simulink model "OilP_DD"  (R2016b)
settings: configuration reference "CodeGenConfigSet" (kept outside this file)
values from neighbouring files (symbols this model uses):
  Oil_pAnaHi_C = Calibration.Parameter    [init_OilP_DD.m]    (also in init_OilP_DD_SIL.m = Simulink.Parameter)
  Oil_pMaxP_CUR = Calibration.Parameter    [init_OilP_DD.m]    (also in init_OilP_DD_SIL.m = Simulink.Parameter)
  Oil_pMaxP_CURX = Calibration.Parameter    [init_OilP_DD.m]    (also in init_OilP_DD_SIL.m = Simulink.Parameter)
  Oil_pMinP_CUR = Calibration.Parameter    [init_OilP_DD.m]    (also in init_OilP_DD_SIL.m = Simulink.Parameter)
  Oil_pMinP_CURX = Calibration.Parameter    [init_OilP_DD.m]    (also in init_OilP_DD_SIL.m = Simulink.Parameter)
  Oil_pTransfPSwmp_CUR = Calibration.Parameter    [init_OilP_DD.m]    (also in init_OilP_DD_SIL.m = Simulink.Parameter)
  Oil_pTransfPSwmp_CURX = Calibration.Parameter    [init_OilP_DD.m]    (also in init_OilP_DD_SIL.m = Simulink.Parameter)
  Oil_tiPhysRngHiPSwmpDefDeb_C = Calibration.Parameter    [init_OilP_DD.m]    (also in init_OilP_DD_SIL.m = Simulink.Parameter)
  Oil_tiPhysRngHiPSwmpOKDeb_C = Calibration.Parameter    [init_OilP_DD.m]    (also in init_OilP_DD_SIL.m = Simulink.Parameter)
  Oil_tiPhysRngLoPSwmpDefDeb_C = Calibration.Parameter    [init_OilP_DD.m]    (also in init_OilP_DD_SIL.m = Simulink.Parameter)
  Oil_tiPhysRngLoPSwmpOKDeb_C = Calibration.Parameter    [init_OilP_DD.m]    (also in init_OilP_DD_SIL.m = Simulink.Parameter)
  Oil_tiSRCMaxPSwmpDefDeb_C = Calibration.Parameter    [init_OilP_DD.m]    (also in init_OilP_DD_SIL.m = Simulink.Parameter)
  Oil_tiSRCMaxPSwmpOKDeb_C = Calibration.Parameter    [init_OilP_DD.m]    (also in init_OilP_DD_SIL.m = Simulink.Parameter)
  Oil_tiSRCMinPSwmpDefDeb_C = Calibration.Parameter    [init_OilP_DD.m]    (also in init_OilP_DD_SIL.m = Simulink.Parameter)
  Oil_tiSRCMinPSwmpOKDeb_C = Calibration.Parameter    [init_OilP_DD.m]    (also in init_OilP_DD_SIL.m = Simulink.Parameter)
  Oil_tLimP_C = Calibration.Parameter    [init_OilP_DD.m]    (also in init_OilP_DD_SIL.m = Simulink.Parameter)
  Oil_uSRCPSwmpMax_C = Calibration.Parameter    [init_OilP_DD.m]    (also in init_OilP_DD_SIL.m = Simulink.Parameter)
  Oil_uSRCPSwmpMin_C = Calibration.Parameter    [init_OilP_DD.m]    (also in init_OilP_DD_SIL.m = Simulink.Parameter)
  OilP_tiPlusDebHiLo_C = Calibration.Parameter    [init_OilP_DD.m]    (also in init_OilP_DD_SIL.m = Simulink.Parameter)
  OilP_tiPlusDebLoHi_C = Calibration.Parameter    [init_OilP_DD.m]    (also in init_OilP_DD_SIL.m = Simulink.Parameter)
undefined symbols (not defined in the file or in its folder): CEngDsT_tTransf_CURX, OilP_DD_DT
libraries: CXLib x13
settings Model: Creator=Wollf  LastModifiedBy=xinchangran
settings ConfigSetRef: SourceLocation=Base Workspace

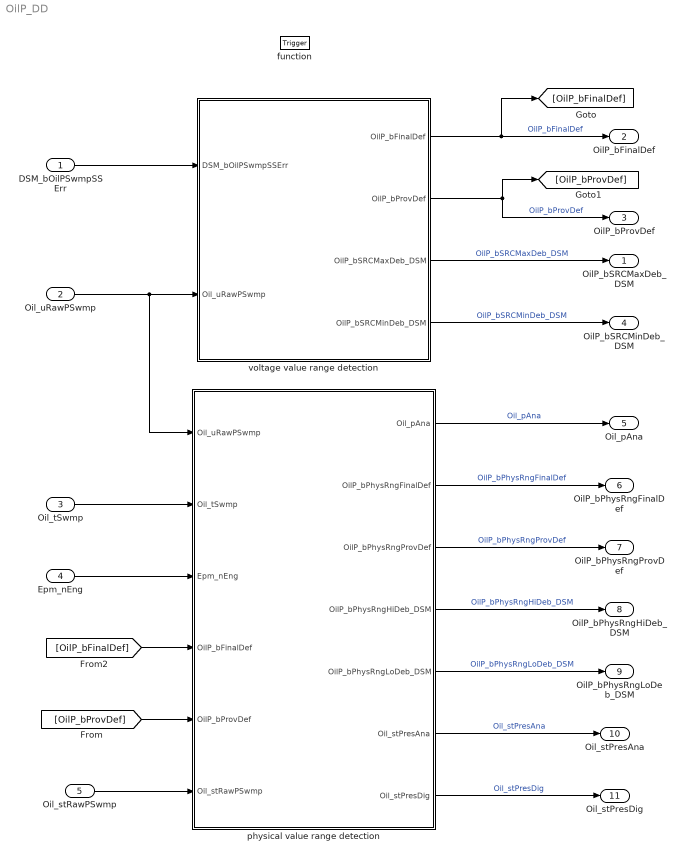
== system OilP_DD ==
  DSM_bOilPSwmpSSErr : Inport  Description=state of FId_OilPSwmpSSErr  OutMin=0  OutMax=1  OutDataTypeStr=boolean
  Oil_uRawPSwmp : Inport  Tag=mv  Description=Raw value of voltage from the ADC  Port=2  OutMin=0  OutMax=5000  OutDataTypeStr=Ad_mv
  Oil_tSwmp : Inport  Tag=deg  Description=Oil temperature in oil sump  Port=3  OutMin=-50  OutMax=200  OutDataTypeStr=Temp_deg
  Epm_nEng : Inport  Tag=rpm  Description=Engine speed  Port=4  OutMin=0  OutMax=6000  OutDataTypeStr=EngSpeed_rpm
  Oil_stRawPSwmp : Inport  Description=the digital sensor raw voltage value  Port=5  OutMin=0  OutMax=1  OutDataTypeStr=boolean
  function : TriggerPort  TriggerType=function-call  VariantControl=Variant
  " voltage value range detection" : Subsystem
  physical value range detection : Subsystem
  OilP_bSRCMaxDeb_DSM : Outport  Description=status of OilP_bSRCMaxDeb  OutMin=0  OutMax=1  OutDataTypeStr=boolean
  OilP_bFinalDef : Outport  Description=Status sensor of the oil pressure finally defect  Port=2  OutMin=0  OutMax=1  OutDataTypeStr=boolean
  OilP_bProvDef : Outport  Description=Status sensor of the oil pressure temporary defect  Port=3  OutMin=0  OutMax=1  OutDataTypeStr=boolean
  OilP_bSRCMinDeb_DSM : Outport  Description=status of OilP_bSRCMinDeb  Port=4  OutMin=0  OutMax=1  OutDataTypeStr=boolean
  Oil_pAna : Outport  Tag=kPa  Description=Oil pressure for analog input  Port=5  OutMin=0  OutMax=1200  OutDataTypeStr=AirPressure_kPa
  OilP_bPhysRngFinalDef : Outport  Description=Status sensor of the oil pressure physical signal range check finally defect  Port=6  OutMin=0  OutMax=1  OutDataTypeStr=boolean
  OilP_bPhysRngProvDef : Outport  Description=Status sensor of the oil pressure physical signal range check temporary defect  Port=7  OutMin=0  OutMax=1  OutDataTypeStr=boolean
  OilP_bPhysRngHiDeb_DSM : Outport  Description=status of OilP_bPhysRngHiDeb  Port=8  OutMin=0  OutMax=1  OutDataTypeStr=boolean
  OilP_bPhysRngLoDeb_DSM : Outport  Description=status of OilP_bPhysRngHiDeb  Port=9  OutMin=0  OutMax=1  OutDataTypeStr=boolean
  Oil_stPresAna : Outport  Description=Oil pressure status for analog input  Port=10  OutMin=0  OutMax=1  OutDataTypeStr=boolean
  Oil_stPresDig : Outport  Description=Oil pressure status for digital input  Port=11  OutMin=0  OutMax=1  OutDataTypeStr=boolean
  wires:
  Oil_uRawPSwmp/1 -> physical value range detection/1(Oil_uRawPSwmp), " voltage value range detection"/2(Oil_uRawPSwmp)
  DSM_bOilPSwmpSSErr/1 -> " voltage value range detection"/1(DSM_bOilPSwmpSSErr)
  " voltage value range detection"/1(OilP_bFinalDef) -> OilP_bFinalDef/1, [OilP_bFinalDef]  "OilP_bFinalDef"
  " voltage value range detection"/2(OilP_bProvDef) -> OilP_bProvDef/1, [OilP_bProvDef]  "OilP_bProvDef"
  " voltage value range detection"/3(OilP_bSRCMaxDeb_DSM) -> OilP_bSRCMaxDeb_DSM/1  "OilP_bSRCMaxDeb_DSM"
  " voltage value range detection"/4(OilP_bSRCMinDeb_DSM) -> OilP_bSRCMinDeb_DSM/1  "OilP_bSRCMinDeb_DSM"
  Oil_tSwmp/1 -> physical value range detection/2(Oil_tSwmp)
  Epm_nEng/1 -> physical value range detection/3(Epm_nEng)
  physical value range detection/1(Oil_pAna) -> Oil_pAna/1  "Oil_pAna"
  physical value range detection/2(OilP_bPhysRngFinalDef) -> OilP_bPhysRngFinalDef/1  "OilP_bPhysRngFinalDef"
  physical value range detection/3(OilP_bPhysRngProvDef) -> OilP_bPhysRngProvDef/1  "OilP_bPhysRngProvDef"
  physical value range detection/4(OilP_bPhysRngHiDeb_DSM) -> OilP_bPhysRngHiDeb_DSM/1  "OilP_bPhysRngHiDeb_DSM"
  physical value range detection/5(OilP_bPhysRngLoDeb_DSM) -> OilP_bPhysRngLoDeb_DSM/1  "OilP_bPhysRngLoDeb_DSM"
  [OilP_bFinalDef] -> physical value range detection/4(OilP_bFinalDef)
  [OilP_bProvDef] -> physical value range detection/5(OilP_bProvDef)
  physical value range detection/6(Oil_stPresAna) -> Oil_stPresAna/1  "Oil_stPresAna"
  physical value range detection/7(Oil_stPresDig) -> Oil_stPresDig/1  "Oil_stPresDig"
  Oil_stRawPSwmp/1 -> physical value range detection/6(Oil_stRawPSwmp)

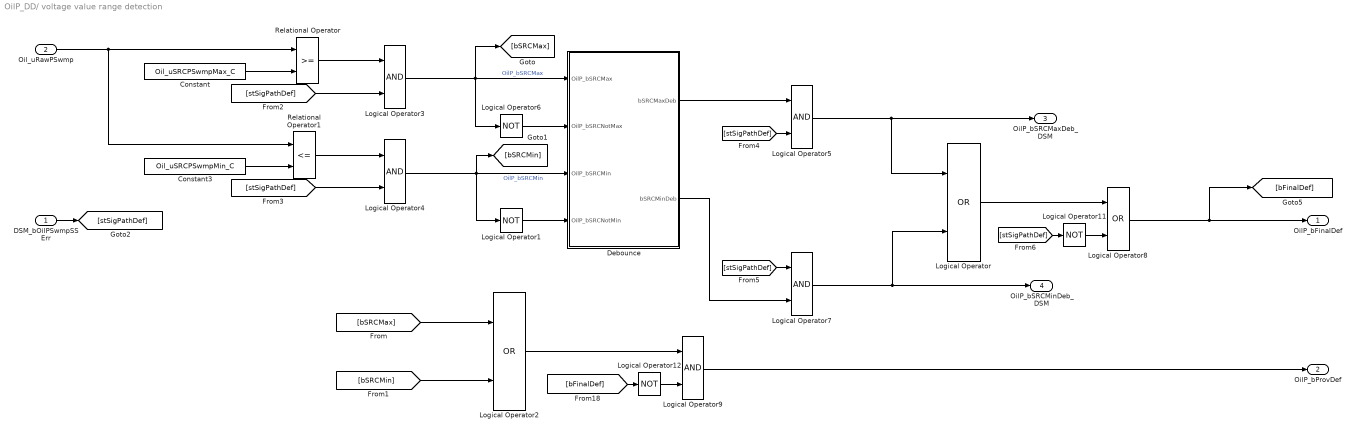
== system OilP_DD/ voltage value range detection ==
  DSM_bOilPSwmpSSErr : Inport
  Oil_uRawPSwmp : Inport  Port=2
  Constant : Constant  Value=Oil_uSRCPSwmpMax_C
  Constant3 : Constant  Value=Oil_uSRCPSwmpMin_C
  Debounce : Subsystem
  Logical Operator : Logic  Operator=OR  AllPortsSameDT=off  OutDataTypeStr=boolean
  Logical Operator{1,6,11..12} (4 alike) : Logic  Operator=NOT  AllPortsSameDT=off  OutDataTypeStr=boolean
  Logical Operator2 : Logic  Operator=OR  AllPortsSameDT=off  OutDataTypeStr=boolean
  Logical Operator{3..5,7,9} (5 alike) : Logic  AllPortsSameDT=off  OutDataTypeStr=boolean
  Logical Operator8 : Logic  Operator=OR  AllPortsSameDT=off  OutDataTypeStr=boolean
  Relational Operator : RelationalOperator  OutDataTypeStr=boolean  RndMeth=Nearest  InputSameDT=on
  Relational Operator1 : RelationalOperator  Operator=<=  OutDataTypeStr=boolean  RndMeth=Nearest  InputSameDT=on
  OilP_bFinalDef : Outport
  OilP_bProvDef : Outport  Port=2
  OilP_bSRCMaxDeb_DSM : Outport  Port=3
  OilP_bSRCMinDeb_DSM : Outport  Port=4
  wires:
  Oil_uRawPSwmp/1 -> Relational Operator1/1, Relational Operator/1
  Relational Operator1/1 -> Logical Operator4/1
  [stSigPathDef] -> Logical Operator3/2
  Logical Operator1/1 -> Debounce/4(OilP_bSRCNotMin)
  Logical Operator12/1 -> Logical Operator9/2
  Debounce/1(bSRCMaxDeb) -> Logical Operator5/1
  Constant/1 -> Relational Operator/2
  [bSRCMin] -> Logical Operator2/2
  Logical Operator4/1 -> [bSRCMin], Debounce/3(OilP_bSRCMin), Logical Operator1/1  "OilP_bSRCMin"
  Logical Operator5/1 -> OilP_bSRCMaxDeb_DSM/1, Logical Operator/1
  [stSigPathDef] -> Logical Operator4/2
  Logical Operator8/1 -> OilP_bFinalDef/1, [bFinalDef]
  Logical Operator7/1 -> OilP_bSRCMinDeb_DSM/1, Logical Operator/2
  Logical Operator9/1 -> OilP_bProvDef/1
  Relational Operator/1 -> Logical Operator3/1
  Logical Operator11/1 -> Logical Operator8/2
  [stSigPathDef] -> Logical Operator5/2
  Logical Operator2/1 -> Logical Operator9/1
  [bSRCMax] -> Logical Operator2/1
  Logical Operator3/1 -> [bSRCMax], Logical Operator6/1, Debounce/1(OilP_bSRCMax)  "OilP_bSRCMax"
  [bFinalDef] -> Logical Operator12/1
  Logical Operator6/1 -> Debounce/2(OilP_bSRCNotMax)
  Debounce/2(bSRCMinDeb) -> Logical Operator7/2
  [stSigPathDef] -> Logical Operator11/1
  Logical Operator/1 -> Logical Operator8/1
  [stSigPathDef] -> Logical Operator7/1
  Constant3/1 -> Relational Operator1/2
  DSM_bOilPSwmpSSErr/1 -> [stSigPathDef]

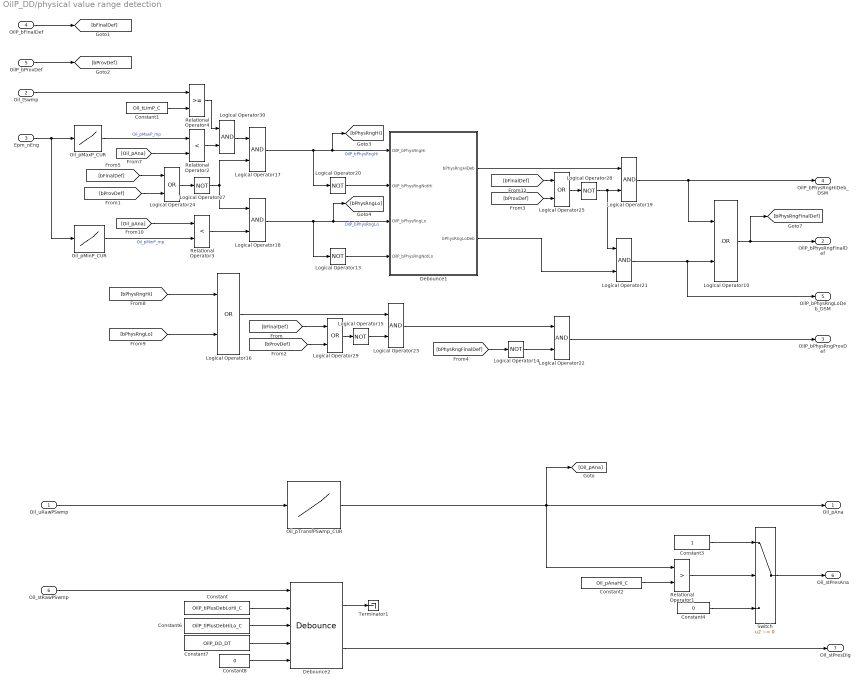
== system OilP_DD/physical value range detection ==
  Oil_uRawPSwmp : Inport
  Oil_tSwmp : Inport  Port=2
  Epm_nEng : Inport  Port=3
  OilP_bFinalDef : Inport  Port=4
  OilP_bProvDef : Inport  Port=5
  Oil_stRawPSwmp : Inport  Port=6
  Constant : Constant  Value=OilP_tiPlusDebLoHi_C
  Constant1 : Constant  Value=Oil_tLimP_C  SampleTime=-1
  Constant2 : Constant  Value=Oil_pAnaHi_C
  Constant3 : Constant  OutDataTypeStr=Inherit: Inherit via back propagation
  Constant4 : Constant  Value=0  OutDataTypeStr=Inherit: Inherit via back propagation
  Constant6 : Constant  Value=OilP_tiPlusDebHiLo_C
  Constant7 : Constant  Value=OilP_DD_DT
  Constant8 : Constant  Value=0  OutDataTypeStr=Inherit: Inherit via back propagation
  Debounce1 : Subsystem
  Debounce2 : CXLib/Debounce
  Logical Operator10 : Logic  Operator=OR  AllPortsSameDT=off  OutDataTypeStr=boolean
  Logical Operator{13..15,20,27..28} (6 alike) : Logic  Operator=NOT  AllPortsSameDT=off  OutDataTypeStr=boolean
  Logical Operator16 : Logic  Operator=OR  AllPortsSameDT=off  OutDataTypeStr=boolean
  Logical Operator{17..19,21..23} (6 alike) : Logic  AllPortsSameDT=off  OutDataTypeStr=boolean
  Logical Operator24 : Logic  Operator=OR  OutDataTypeStr=boolean
  Logical Operator25 : Logic  Operator=OR  OutDataTypeStr=boolean
  Logical Operator29 : Logic  Operator=OR  OutDataTypeStr=boolean
  Logical Operator30 : Logic  OutDataTypeStr=boolean
  Oil_pMaxP_CUR : Lookup_n-D  DialogController=Simulink.DDGSource  NumberOfTableDimensions=1  BreakpointsForDimension1=Oil_pMaxP_CURX  BreakpointsForDimension2=CEngDsT_tTransf_CURX  IndexSearchMethod=Linear search  BeginIndexSearchUsingPreviousIndexResult=on  Table=Oil_pMaxP_CUR  ExtrapMethod=Clip  UseLastTableValue=on  InternalRulePriority=Speed  OutDataTypeStr=Inherit: Inherit via back propagation  SaturateOnIntegerOverflow=on
  Oil_pMinP_CUR : Lookup_n-D  DialogController=Simulink.DDGSource  NumberOfTableDimensions=1  BreakpointsForDimension1=Oil_pMinP_CURX  BreakpointsForDimension2=CEngDsT_tTransf_CURX  IndexSearchMethod=Linear search  BeginIndexSearchUsingPreviousIndexResult=on  Table=Oil_pMinP_CUR  ExtrapMethod=Clip  UseLastTableValue=on  InternalRulePriority=Speed  OutDataTypeStr=Inherit: Inherit via back propagation  SaturateOnIntegerOverflow=on
  Oil_pTransfPSwmp_CUR : Lookup_n-D  DialogController=Simulink.DDGSource  NumberOfTableDimensions=1  BreakpointsForDimension1=Oil_pTransfPSwmp_CURX  BreakpointsForDimension2=CEngDsT_tTransf_CURX  IndexSearchMethod=Linear search  BeginIndexSearchUsingPreviousIndexResult=on  Table=Oil_pTransfPSwmp_CUR  ExtrapMethod=Clip  UseLastTableValue=on  InternalRulePriority=Speed  OutDataTypeStr=Inherit: Inherit via back propagation  SaturateOnIntegerOverflow=on
  Relational Operator1 : RelationalOperator  Operator=>  OutDataTypeStr=boolean  RndMeth=Nearest  InputSameDT=on
  Relational Operator2 : RelationalOperator  Operator=<  OutDataTypeStr=boolean  RndMeth=Nearest  InputSameDT=on
  Relational Operator3 : RelationalOperator  Operator=<  OutDataTypeStr=boolean  RndMeth=Nearest  InputSameDT=on
  Relational Operator4 : RelationalOperator  OutDataTypeStr=boolean  RndMeth=Nearest  InputSameDT=on
  Switch : Switch  Criteria=u2 ~= 0  InputSameDT=on
  Terminator1 : Terminator
  Oil_pAna : Outport
  OilP_bPhysRngFinalDef : Outport  Port=2
  OilP_bPhysRngProvDef : Outport  Port=3
  OilP_bPhysRngHiDeb_DSM : Outport  Port=4
  OilP_bPhysRngLoDeb_DSM : Outport  Port=5
  Oil_stPresAna : Outport  Port=6
  Oil_stPresDig : Outport  Port=7
  wires:
  Logical Operator17/1 -> Logical Operator20/1, Debounce1/1(OilP_bPhysRngHi), [bPhysRngHi]  "OilP_bPhysRngHi"
  Logical Operator18/1 -> Logical Operator13/1, [bPhysRngLo], Debounce1/3(OilP_bPhysRngLo)  "OilP_bPhysRngLo"
  Oil_pMinP_CUR/1 -> Relational Operator3/2  "Oil_pMinP_mp"
  [bPhysRngHi] -> Logical Operator16/1
  [bPhysRngLo] -> Logical Operator16/2
  Logical Operator24/1 -> Logical Operator27/1
  Logical Operator21/1 -> OilP_bPhysRngLoDeb_DSM/1, Logical Operator10/2
  Logical Operator22/1 -> OilP_bPhysRngProvDef/1
  Relational Operator4/1 -> Logical Operator30/1
  Logical Operator28/1 -> Logical Operator21/1, Logical Operator19/2
  Logical Operator20/1 -> Debounce1/2(OilP_bPhysRngNotHi)
  [bProvDef] -> Logical Operator24/2
  Logical Operator29/1 -> Logical Operator15/1
  [bFinalDef] -> Logical Operator24/1
  Epm_nEng/1 -> Oil_pMinP_CUR/1, Oil_pMaxP_CUR/1
  Relational Operator2/1 -> Logical Operator30/2
  Logical Operator10/1 -> OilP_bPhysRngFinalDef/1, [bPhysRngFinalDef]
  Logical Operator30/1 -> Logical Operator17/1
  Debounce1/2(bPhysRngLoDeb) -> Logical Operator21/2
  Constant1/1 -> Relational Operator4/2
  [bPhysRngFinalDef] -> Logical Operator14/1
  [bProvDef] -> Logical Operator25/2
  Logical Operator14/1 -> Logical Operator22/2
  [bFinalDef] -> Logical Operator29/1
  Oil_tSwmp/1 -> Relational Operator4/1
  [bFinalDef] -> Logical Operator25/1
  Logical Operator25/1 -> Logical Operator28/1
  Oil_pMaxP_CUR/1 -> Relational Operator2/1  "Oil_pMaxP_mp"
  [bProvDef] -> Logical Operator29/2
  Logical Operator27/1 -> Logical Operator18/1, Logical Operator17/2
  Logical Operator23/1 -> Logical Operator22/1
  Logical Operator16/1 -> Logical Operator23/1
  Logical Operator15/1 -> Logical Operator23/2
  Debounce1/1(bPhysRngHiDeb) -> Logical Operator19/1
  Relational Operator3/1 -> Logical Operator18/2
  Logical Operator13/1 -> Debounce1/4(OilP_bPhysRngNotLo)
  Oil_uRawPSwmp/1 -> Oil_pTransfPSwmp_CUR/1
  OilP_bProvDef/1 -> [bProvDef]
  OilP_bFinalDef/1 -> [bFinalDef]
  [Oil_pAna] -> Relational Operator2/2
  [Oil_pAna] -> Relational Operator3/1
  Constant2/1 -> Relational Operator1/2
  Relational Operator1/1 -> Switch/2
  Constant3/1 -> Switch/1
  Constant4/1 -> Switch/3
  Switch/1 -> Oil_stPresAna/1
  Constant6/1 -> Debounce2/3
  Debounce2/1 -> Terminator1/1
  Constant/1 -> Debounce2/2
  Constant7/1 -> Debounce2/4
  Constant8/1 -> Debounce2/5
  Oil_stRawPSwmp/1 -> Debounce2/1
  Debounce2/2 -> Oil_stPresDig/1
  Oil_pTransfPSwmp_CUR/1 -> [Oil_pAna], Oil_pAna/1, Relational Operator1/1
  Logical Operator19/1 -> OilP_bPhysRngHiDeb_DSM/1, Logical Operator10/1

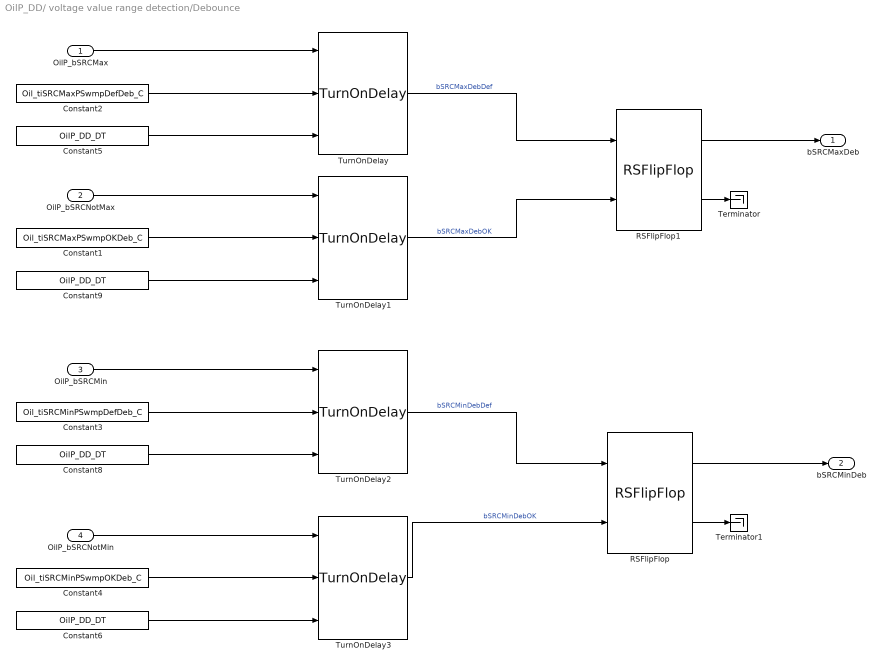
== system OilP_DD/ voltage value range detection/Debounce ==
  OilP_bSRCMax : Inport
  OilP_bSRCNotMax : Inport  Port=2
  OilP_bSRCMin : Inport  Port=3
  OilP_bSRCNotMin : Inport  Port=4
  Constant1 : Constant  Value=Oil_tiSRCMaxPSwmpOKDeb_C
  Constant2 : Constant  Value=Oil_tiSRCMaxPSwmpDefDeb_C
  Constant3 : Constant  Value=Oil_tiSRCMinPSwmpDefDeb_C
  Constant4 : Constant  Value=Oil_tiSRCMinPSwmpOKDeb_C
  Constant{5..6,8..9} (4 alike) : Constant  Value=OilP_DD_DT  OutDataTypeStr=Inherit: Inherit via back propagation
  RSFlipFlop : CXLib/RSFlipFlop
  RSFlipFlop1 : CXLib/RSFlipFlop
  Terminator : Terminator
  Terminator1 : Terminator
  TurnOnDelay{,1..3} (4 alike) : CXLib/TurnOnDelay
  bSRCMaxDeb : Outport
  bSRCMinDeb : Outport  Port=2
  wires:
  RSFlipFlop/1 -> bSRCMinDeb/1
  RSFlipFlop1/1 -> bSRCMaxDeb/1
  TurnOnDelay1/1 -> RSFlipFlop1/2  "bSRCMaxDebOK"
  Constant3/1 -> TurnOnDelay2/2
  Constant1/1 -> TurnOnDelay1/2
  Constant2/1 -> TurnOnDelay/2
  TurnOnDelay/1 -> RSFlipFlop1/1  "bSRCMaxDebDef"
  OilP_bSRCNotMax/1 -> TurnOnDelay1/1
  OilP_bSRCMin/1 -> TurnOnDelay2/1
  TurnOnDelay2/1 -> RSFlipFlop/1  "bSRCMinDebDef"
  OilP_bSRCNotMin/1 -> TurnOnDelay3/1
  TurnOnDelay3/1 -> RSFlipFlop/2  "bSRCMinDebOK"
  Constant4/1 -> TurnOnDelay3/2
  RSFlipFlop1/2 -> Terminator/1
  RSFlipFlop/2 -> Terminator1/1
  OilP_bSRCMax/1 -> TurnOnDelay/1
  Constant5/1 -> TurnOnDelay/3
  Constant8/1 -> TurnOnDelay2/3
  Constant6/1 -> TurnOnDelay3/3
  Constant9/1 -> TurnOnDelay1/3

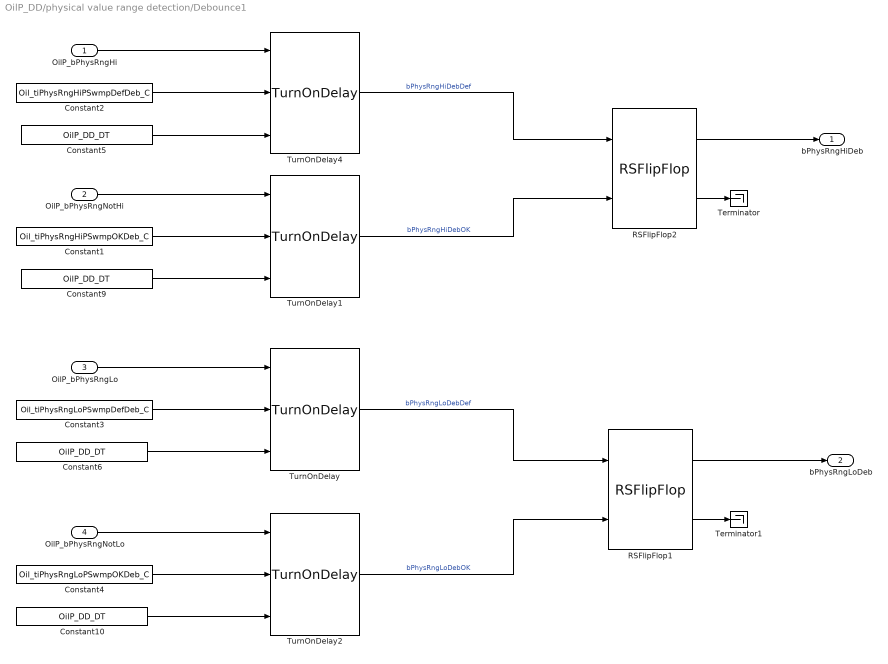
== system OilP_DD/physical value range detection/Debounce1 ==
  OilP_bPhysRngHi : Inport
  OilP_bPhysRngNotHi : Inport  Port=2
  OilP_bPhysRngLo : Inport  Port=3
  OilP_bPhysRngNotLo : Inport  Port=4
  Constant1 : Constant  Value=Oil_tiPhysRngHiPSwmpOKDeb_C
  Constant{5..6,9..10} (4 alike) : Constant  Value=OilP_DD_DT  OutDataTypeStr=Inherit: Inherit via back propagation
  Constant2 : Constant  Value=Oil_tiPhysRngHiPSwmpDefDeb_C
  Constant3 : Constant  Value=Oil_tiPhysRngLoPSwmpDefDeb_C
  Constant4 : Constant  Value=Oil_tiPhysRngLoPSwmpOKDeb_C
  RSFlipFlop1 : CXLib/RSFlipFlop
  RSFlipFlop2 : CXLib/RSFlipFlop
  Terminator : Terminator
  Terminator1 : Terminator
  TurnOnDelay{,1..2,4} (4 alike) : CXLib/TurnOnDelay
  bPhysRngHiDeb : Outport
  bPhysRngLoDeb : Outport  Port=2
  wires:
  OilP_bPhysRngHi/1 -> TurnOnDelay4/1
  RSFlipFlop1/2 -> Terminator1/1
  RSFlipFlop2/2 -> Terminator/1
  Constant4/1 -> TurnOnDelay2/2
  TurnOnDelay2/1 -> RSFlipFlop1/2  "bPhysRngLoDebOK"
  OilP_bPhysRngNotLo/1 -> TurnOnDelay2/1
  TurnOnDelay/1 -> RSFlipFlop1/1  "bPhysRngLoDebDef"
  OilP_bPhysRngLo/1 -> TurnOnDelay/1
  OilP_bPhysRngNotHi/1 -> TurnOnDelay1/1
  TurnOnDelay4/1 -> RSFlipFlop2/1  "bPhysRngHiDebDef"
  Constant2/1 -> TurnOnDelay4/2
  Constant1/1 -> TurnOnDelay1/2
  Constant3/1 -> TurnOnDelay/2
  TurnOnDelay1/1 -> RSFlipFlop2/2  "bPhysRngHiDebOK"
  RSFlipFlop2/1 -> bPhysRngHiDeb/1
  RSFlipFlop1/1 -> bPhysRngLoDeb/1
  Constant5/1 -> TurnOnDelay4/3
  Constant9/1 -> TurnOnDelay1/3
  Constant6/1 -> TurnOnDelay/3
  Constant10/1 -> TurnOnDelay2/3
